simulink model "MPC_Pseudostates"  (R2020a)
settings: Solver=VariableStepAuto  StartTime=0.0  StopTime=5  RelTol=1e-3
values from neighbouring files (symbols this model uses):
  l = 0.25    [init.m]    (also in matlab.mat)
libraries: mpclib x1, cstblocks x1

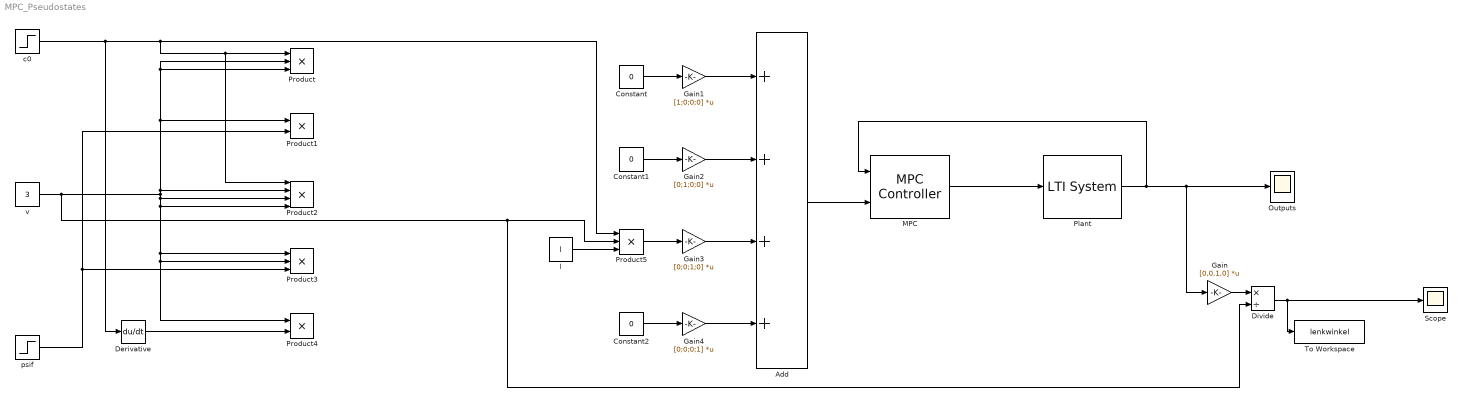
== system MPC_Pseudostates ==
  Add : Sum  Inputs=++++
  Constant : Constant  Value=0
  Constant1 : Constant  Value=0
  Constant2 : Constant  Value=0
  Derivative : Derivative
  Divide : Product  Inputs=*/
  Gain : Gain  Gain=[0,0,1,0]  Multiplication=Matrix(K*u)
  Gain1 : Gain  Gain=[1;0;0;0]  Multiplication=Matrix(K*u)
  Gain2 : Gain  Gain=[0;1;0;0]  Multiplication=Matrix(K*u)
  Gain3 : Gain  Gain=[0;0;1;0]  Multiplication=Matrix(K*u)
  Gain4 : Gain  Gain=[0;0;0;1]  Multiplication=Matrix(K*u)
  MPC : mpclib/MPC Controller  SCDEnableBlockLinearizationSpecification=on  mpcobj=mpc1_1_C_2  is_multiple=0  enable_value=0  return_u0=off  updateMPCinCallerWorkspace=on  md_inport=off  mv_inport=off  uref_inport=off  return_cost=off  return_mvseq=off  return_qpstatus=off  return_xseq=off  return_state=off  return_ovseq=off  state_inport=off  umin_inport=off  umax_inport=off  ymin_inport=off  ymax_inport=off  cc_inport=off  ywt_inport=off  uwt_inport=off  duwt_inport=off  rhoeps_inport=off  pm_inport=off  MaximumP=10  HorizonChoice=FixedHorizon  n_ts=0.05  n_p=10  n_mv=5  n_md=0  n_ud=0  n_mo=4  n_uo=0  BlockDataType=double  SampleTimeInherited=off  switch_inport=off
  Outputs : Scope
  Plant : cstblocks/LTI System  sys=mpc1_1_G_2  IC=[]
  Product : Product  Inputs=3
  Product1 : Product
  Product2 : Product  Inputs=4
  Product3 : Product  Inputs=3
  Product4 : Product
  Product5 : Product  Inputs=3
  Scope : Scope
  To Workspace : ToWorkspace  VariableName=lenkwinkel  SaveFormat=Timeseries  SampleTime=-1
  c0 : Step  SampleTime=0
  l : Constant  Value=l
  psif : Step  After=0.5  SampleTime=0
  v : Constant  Value=3
  wires:
  Plant/1 -> MPC/1, Gain/1, Outputs/1
  MPC/1 -> Plant/1
  Add/1 -> MPC/2
  Gain1/1 -> Add/1
  Gain4/1 -> Add/4
  Gain3/1 -> Add/3
  Gain2/1 -> Add/2
  c0/1 -> Product5/1, Product2/1, Product/1, Derivative/1
  v/1 -> Divide/2, Product5/2, Product4/1, Product3/2, Product3/1, Product2/4, Product2/3, Product2/2, Product1/1, Product/2, Product/3
  psif/1 -> Product3/3, Product1/2
  Derivative/1 -> Product4/2
  Constant/1 -> Gain1/1
  Constant1/1 -> Gain2/1
  Product5/1 -> Gain3/1
  l/1 -> Product5/3
  Constant2/1 -> Gain4/1
  Gain/1 -> Divide/1
  Divide/1 -> To Workspace/1, Scope/1
